simulink model "hoop_pose_2021"  (R2022a)
settings: Solver=VariableStepAuto  StartTime=0.0  StopTime=10.0  RelTol=1e-3
libraries: robotlib x5
settings Model: Creator=cftemp3  LastModifiedBy=dtu31390
settings DebuggingCC: UnconnectedInputMsg=warning  UnconnectedOutputMsg=warning  UnconnectedLineMsg=warning
settings RTWCC: DLArmComputeVersion=19.05

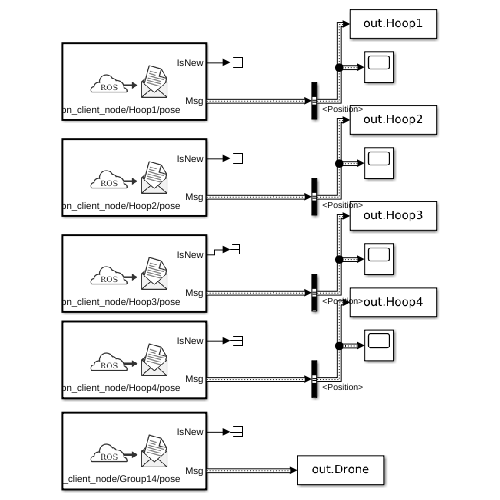
[thumbnail: Simulink's stored preview of the top-level diagram]
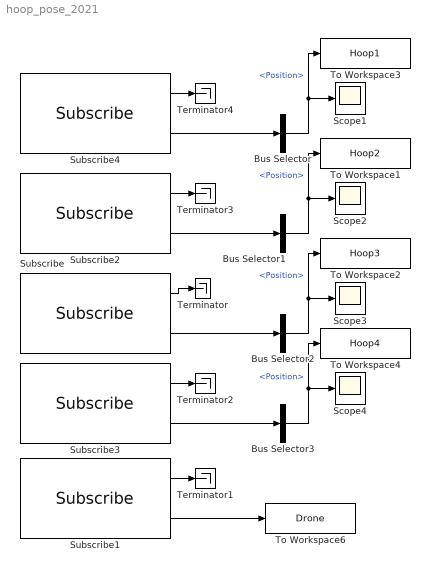
== system hoop_pose_2021 ==
  Bus Selector{,1..3} (4 alike) : BusSelector  OutputSignals=Pose.Position
  Scope{1..4} (4 alike) : Scope
  Subscribe : robotlib/Subscribe  topicSource=Select from ROS network  topic=/vrpn_client_node/Hoop3/pose  messageType=geometry_msgs/PoseStamped  SampleTime=-1  legacyBusStruct=off  messageQueueLength=1
  Subscribe1 : robotlib/Subscribe  topicSource=Select from ROS network  topic=/vrpn_client_node/Group14/pose  messageType=geometry_msgs/PoseStamped  SampleTime=-1  legacyBusStruct=off  messageQueueLength=1
  Subscribe2 : robotlib/Subscribe  topicSource=Select from ROS network  topic=/vrpn_client_node/Hoop2/pose  messageType=geometry_msgs/PoseStamped  SampleTime=-1  legacyBusStruct=off  messageQueueLength=1
  Subscribe3 : robotlib/Subscribe  topicSource=Select from ROS network  topic=/vrpn_client_node/Hoop4/pose  messageType=geometry_msgs/PoseStamped  SampleTime=-1  legacyBusStruct=off  messageQueueLength=1
  Subscribe4 : robotlib/Subscribe  topicSource=Select from ROS network  topic=/vrpn_client_node/Hoop1/pose  messageType=geometry_msgs/PoseStamped  SampleTime=-1  legacyBusStruct=off  messageQueueLength=1
  Terminator{,1..4} (5 alike) : Terminator
  To Workspace1 : ToWorkspace  VariableName=Hoop2  SaveFormat=Timeseries  SampleTime=-1
  To Workspace2 : ToWorkspace  VariableName=Hoop3  SaveFormat=Timeseries  SampleTime=-1
  To Workspace3 : ToWorkspace  VariableName=Hoop1  SaveFormat=Timeseries  SampleTime=-1
  To Workspace4 : ToWorkspace  VariableName=Hoop4  SaveFormat=Timeseries  SampleTime=-1
  To Workspace6 : ToWorkspace  VariableName=Drone  SaveFormat=Timeseries  SampleTime=-1
  wires:
  Subscribe4/2 -> Bus Selector/1
  Subscribe1/1 -> Terminator1/1
  Subscribe3/1 -> Terminator2/1
  Subscribe/1 -> Terminator/1
  Subscribe2/1 -> Terminator3/1
  Subscribe4/1 -> Terminator4/1
  Bus Selector/1 -> To Workspace3/1, Scope1/1  "<Position>"
  Bus Selector1/1 -> To Workspace1/1, Scope2/1  "<Position>"
  Subscribe2/2 -> Bus Selector1/1
  Bus Selector2/1 -> To Workspace2/1, Scope3/1  "<Position>"
  Bus Selector3/1 -> To Workspace4/1, Scope4/1  "<Position>"
  Subscribe3/2 -> Bus Selector3/1
  Subscribe1/2 -> To Workspace6/1
  Subscribe/2 -> Bus Selector2/1
